simulink model "LQR_sim_lin"  (R2016b)
settings: Solver=VariableStepAuto  StartTime=0.0  StopTime=20  FixedStep=Ts  RelTol=1e-3
values from neighbouring files (symbols this model uses):
  A_0 = [0 -3.26931291643 0 0.71460251427 0 0 0 0 1 -0.0325743287495 0 -0.000548520916999 ... (64 elements, 8x8)]    [parametros.mat]    (also in twin_rotor_modelo_V1.m = eval(A_0))
  B_0 = [0 0 0 0 0 0 1190.47619048 0 0 0 0 0 ... (16 elements, 8x2)]    [parametros.mat]    (also in twin_rotor_modelo_V1.m = eval(B_0))
  C_0 = [1 0 0 0 0 1 0 0 0 0 0 0 ... (16 elements, 2x8)]    [parametros.mat]    (also in twin_rotor_modelo_V1.m = eval(C_0))
undefined symbols (not defined in the file or in its folder): K
settings Model: Creator=cristobal  LastModifiedBy=cristobal

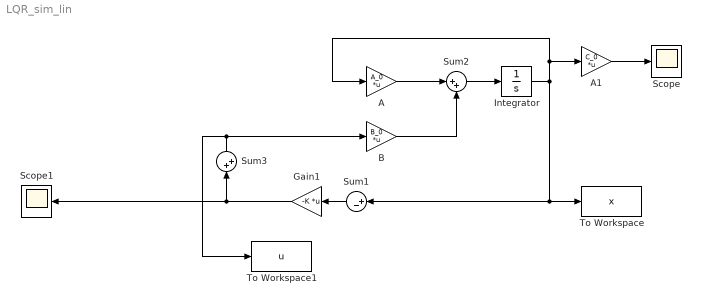
== system LQR_sim_lin ==
  A : Gain  Gain=A_0  Multiplication=Matrix(K*u)
  A1 : Gain  Gain=C_0  Multiplication=Matrix(K*u)
  B : Gain  Gain=B_0  Multiplication=Matrix(K*u)
  Gain1 : Gain  Gain=-K  Multiplication=Matrix(K*u)
  Integrator : Integrator  InitialCondition=ci'
  Scope : Scope
  Scope1 : Scope
  Sum1 : Sum  Inputs=|+-
  Sum2 : Sum  Inputs=|++
  Sum3 : Sum  Inputs=|++
  To Workspace : ToWorkspace  VariableName=x  SaveFormat=Timeseries  SampleTime=-1
  To Workspace1 : ToWorkspace  VariableName=u  SaveFormat=Timeseries  SampleTime=-1
  wires:
  Sum1/1 -> Gain1/1
  A/1 -> Sum2/1
  B/1 -> Sum2/2
  Sum2/1 -> Integrator/1
  Integrator/1 -> A1/1, A/1, To Workspace/1, Sum1/1
  Gain1/1 -> Sum3/1, Scope1/1
  A1/1 -> Scope/1
  Sum3/1 -> B/1, To Workspace1/1
